simulink model "SnapshotTestBench"  (R2024b)
settings: Solver=VariableStepAuto  StartTime=0.0  StopTime=scenario.StopTime  FixedStep=Ts  RelTol=1e-3
PostLoadFcn:
  | clear all
  | helperSLHighwayLaneChangePlannerSetup
values from neighbouring files (symbols this model uses):
  egoInitialPose = evalin('base','egoInitialPose')    [HelperPlotLCPlannerStatus.m]    (also in HelperPlotLCPlannerStatus_RMC.m; helperSLHighwayLaneChangePlannerSetup.m = struct('ActorID', EgoActor.ActorID,                         )
  mapInfo = struct('NumLanes', numLanes,'LaneWidth', zeros(maxNumLanes,1),                  'LaneCenters', zeros(maxNumLanes,1),'NumGlobalPlanPoints',                  size(globalPlanPoints,1), 'GlobalPlanPoints',                  zeros(maxGlobalPlanPoints,2), 'LaneLateralBoundary', zeros(maxNumLanes, 2))    [helperSLHighwayLaneChangePlannerSetup.m]
  replanRate = 1    [helperSLHighwayLaneChangePlannerSetup.m]
  timeHorizon = 1:3    [helperSLHighwayLaneChangePlannerSetup.m]
  timeResolution = 0.1    [helperSLHighwayLaneChangePlannerSetup.m]
  velocityHorizon = 2    [helperSLHighwayLaneChangePlannerSetup.m]
undefined symbols (not defined in the file or in its folder): ActorID, actorProfiles, AngularVelocity, assessment, egoFrontExt, egoTTC, enableCCBehavior, enableLCBehavior, enableLCFBehavior, frontSafetyGap, latDevCost, maxAccel, maxCurvature, maxPlanningHorizon, maxYawRate, minVelocity, nextTTC, Position, preferredLane, rearSafetyGap, setSpeed, speedCost, targetFrontExt, timeCost, Ts, Velocity, Yaw
libraries: simulink x7, drivingscenarioandsensors x2
CloseFcn:
  | helperSLHighwayLaneChangePlannerCleanUp
settings Model: Creator=The MathWorks, Inc.  LastModifiedBy=grape
settings SolverCC: ZeroCrossAlgorithm=Adaptive  AlgebraicLoopSolver=TrustRegion  MaxZcPerStep=1
settings DataIOCC: SaveOutput=off  ReturnWorkspaceOutputs=off
settings OptimizationCC: ReuseModelBlockBuffer=off  ZeroExternalMemoryAtStartup=off  ZeroInternalMemoryAtStartup=off  OptimizeBlockOrder=speed
settings DebuggingCC: MaskedZcDiagnostic=none  IgnoredZcDiagnostic=none  UnconnectedInputMsg=warning  UnconnectedOutputMsg=warning  UnconnectedLineMsg=warning  SubsystemReferenceDiagnosticForUnitTest=warning
settings ModelReferenceCC: EnableRefExpFcnMdlSchedulingChecks=on
settings RTWCC: Description=Embedded Coder  SystemTargetFile=ert.tlc  TemplateMakefile=ert_default_tmf  PortableWordSizes=on  CodeProfilingSaveOptions=AllData  TargetLang=C++  GPUComputeCapability=3.5  DLArmComputeVersion=19.05
settings CodeAppCC: ForceParamTrailComments=on  IgnoreCustomStorageClasses=off  OperatorAnnotations=on  SimulinkDataObjDesc=on  SFDataObjDesc=on  InsertBlockDesc=on
settings ERTTargetCC: TargetLangStandard=C++03 (ISO)  GenerateSampleERTMain=on  CodeInterfacePackaging=C++ class  InlinedParameterPlacement=Hierarchical  RootIOFormat=Structure reference  ERTCustomFileTemplate=example_file_process.tlc  DynamicArrayContainerType=coder::array
settings ConfigComp: CovScope=ReferencedModels  CovIncludeTopModel=off  CovMetricSettings=dtrzoibwe

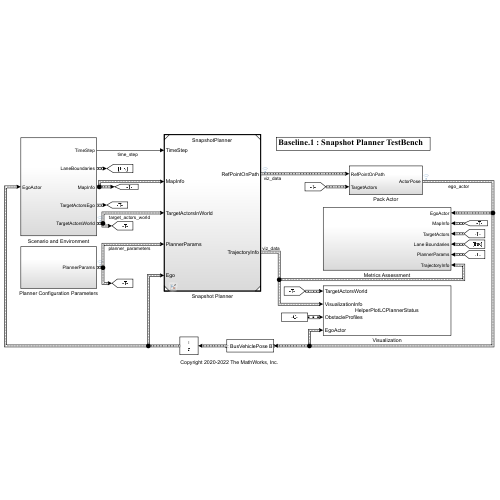
[thumbnail: Simulink's stored preview of the top-level diagram]
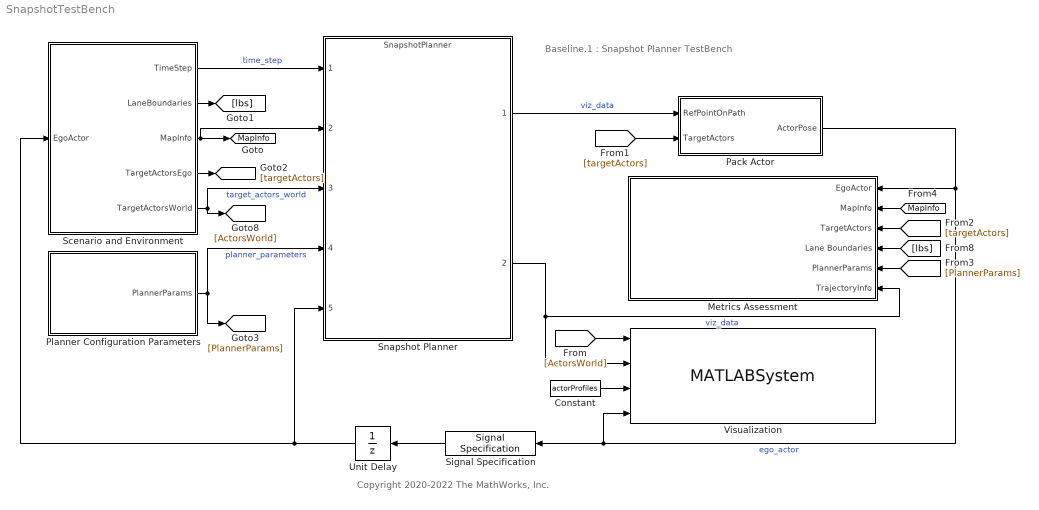
== system SnapshotTestBench ==
  note: Baseline.1 : Snapshot Planner TestBench
  note: Copyright 2020-2022 The MathWorks, Inc.
  Constant : Constant  Value=actorProfiles  OutDataTypeStr=Bus: BusActorProfiles
  Metrics Assessment : Subsystem
  Pack Actor : Subsystem
  Planner Configuration Parameters : Subsystem
  Scenario and Environment : Subsystem
  Signal Specification : SignalSpecification  OutDataTypeStr=Bus: BusVehiclePose  BusOutputAsStruct=on
  Snapshot Planner : ModelReference  ModelNameDialog=SnapshotPlanner.slx  SimulationMode=Normal  ModelReferenceVersion=10.9
  Unit Delay : UnitDelay  InitialCondition=egoInitialPose  SampleTime=-1  HasFrameUpgradeWarning=on
  Visualization : MATLABSystem  System=HelperPlotLCPlannerStatus  EnableTopView=on  EnableTrajTopView=on  EnableChaseView=on  EnableTrajChase=on  EnableCaplistChaseView=on
      mask Type: HelperPlotLCPlannerStatus
      mask Display:
      | disp('HelperPlotLCPlannerStatus');
      | port_label('input',1,'TargetActorsWorld');
      | port_label('input',2,'VisualizationInfo');
      | port_label('input',3,'ObstacleProfiles');
      | port_label('input',4,'EgoActor');
  tag scope: MapInfo=global
  wires:
  Scenario and Environment/4(TargetActorsEgo) -> [targetActors]
  Scenario and Environment/2(LaneBoundaries) -> [lbs]
  Signal Specification/1 -> Unit Delay/1
  [targetActors] -> Pack Actor/2(TargetActors)
  Scenario and Environment/5(TargetActorsWorld) -> Snapshot Planner/3, [ActorsWorld]  "target_actors_world"
  Scenario and Environment/3(MapInfo) -> Snapshot Planner/2, [MapInfo]
  Constant/1 -> Visualization/3
  [ActorsWorld] -> Visualization/1
  Planner Configuration Parameters/1(PlannerParams) -> [PlannerParams], Snapshot Planner/4  "planner_parameters"
  Pack Actor/1(ActorPose) -> Metrics Assessment/1(EgoActor), Visualization/4, Signal Specification/1  "ego_actor"
  Snapshot Planner/2 -> Metrics Assessment/6(TrajectoryInfo), Visualization/2  "viz_data"
  Scenario and Environment/1(TimeStep) -> Snapshot Planner/1  "time_step"
  [targetActors] -> Metrics Assessment/3(TargetActors)
  [lbs] -> Metrics Assessment/4(Lane Boundaries)
  [PlannerParams] -> Metrics Assessment/5(PlannerParams)
  [MapInfo] -> Metrics Assessment/2(MapInfo)
  Snapshot Planner/1 -> Pack Actor/1(RefPointOnPath)  "viz_data"
  Unit Delay/1 -> Scenario and Environment/1(EgoActor), Snapshot Planner/5

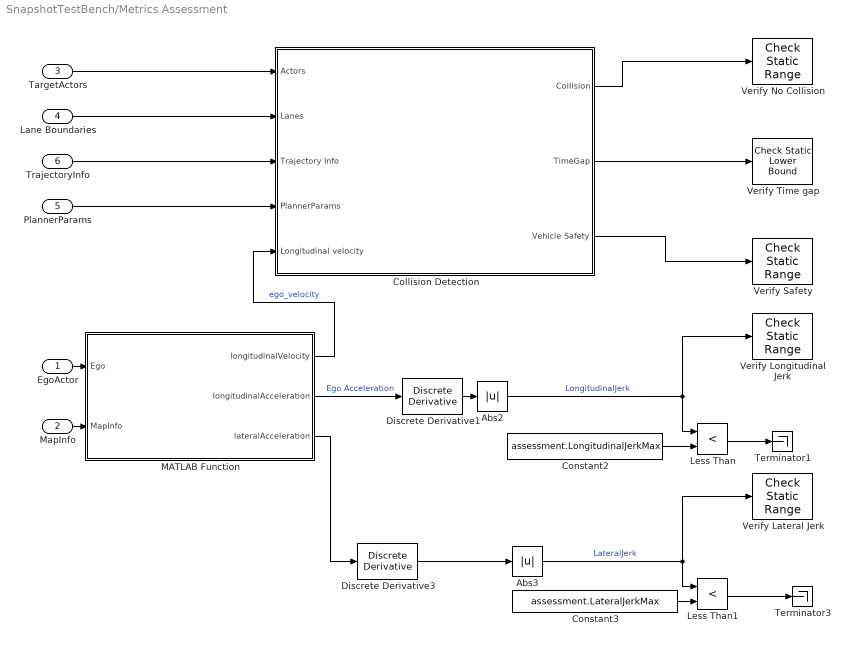
== system SnapshotTestBench/Metrics Assessment ==
  EgoActor : Inport
  MapInfo : Inport  Port=2
  TargetActors : Inport  Port=3
  Lane Boundaries : Inport  Port=4
  PlannerParams : Inport  Port=5
  TrajectoryInfo : Inport  Port=6
  Abs2 : Abs  ZeroCross=off  SaturateOnIntegerOverflow=off
  Abs3 : Abs  ZeroCross=off  SaturateOnIntegerOverflow=off
  Collision Detection : Subsystem
  Constant2 : Constant  Value=assessment.LongitudinalJerkMax
  Constant3 : Constant  Value=assessment.LateralJerkMax
  Discrete Derivative1 : simulink/Discrete/Discrete Derivative  gainval=0.1  ICPrevScaledInput=0.1/Ts  OutMin=[]  OutMax=[]  OutDataType=fixdt(1, 16)  OutScaling=2^-10  DoSatur=off
  Discrete Derivative3 : simulink/Discrete/Discrete Derivative  gainval=0.1  ICPrevScaledInput=0.1/Ts  OutMin=[]  OutMax=[]  OutDataType=fixdt(1, 16)  OutScaling=2^-10  DoSatur=off
  Less Than : RelationalOperator  Operator=<  OutDataTypeStr=boolean  RndMeth=Simplest  InputSameDT=off
  Less Than1 : RelationalOperator  Operator=<  OutDataTypeStr=boolean  RndMeth=Simplest  InputSameDT=off
  MATLAB Function : MATLAB Function  TreatAsAtomicUnit=on
  Terminator1 : Terminator
  Terminator3 : Terminator
  Verify Lateral Jerk : simulink/Model Verification/Check  Static Range  Description=-assessment.LateralJerkMax <= u <= assessment.LateralJerkMax  max=assessment.LateralJerkMax  max_included=on  min=-assessment.LateralJerkMax  min_included=on  enabled=on  stopWhenAssertionFail=off  export=off  icon=graphic
      settings: AttributesFormatString=|
      | ---------------------------------------
      | max = %<max>
      | min = %<min>
  Verify Longitudinal Jerk : simulink/Model Verification/Check  Static Range  Description=-assessment.LongitudinalJerkMax <= u <= assessment.LongitudinalJerkMax  max=assessment.LongitudinalJerkMax  max_included=on  min=-assessment.LongitudinalJerkMax  min_included=on  enabled=on  stopWhenAssertionFail=off  export=off  icon=graphic
      settings: AttributesFormatString=|
      | ---------------------------------------
      | max = %<max>
      | min = %<min>
  Verify No Collision : simulink/Model Verification/Check  Static Range  Description=0 <= u <= 0  max=0  max_included=on  min=0  min_included=on  enabled=on  stopWhenAssertionFail=on  export=off  icon=graphic
  Verify Safety : simulink/Model Verification/Check  Static Range  Description=1 <= u <= 1  max=1  max_included=on  min=1  min_included=on  enabled=on  stopWhenAssertionFail=off  export=off  icon=graphic
  Verify Time gap : simulink/Model Verification/Check Static  Lower Bound  Description=assessment.TimeGap <= u  min=assessment.TimeGap  min_included=on  enabled=on  stopWhenAssertionFail=off  export=off  icon=graphic
      settings: AttributesFormatString=|
      | ---------------------------------------
      | min = %<min>
  wires:
  PlannerParams/1 -> Collision Detection/4(PlannerParams)
  Collision Detection/1(Collision) -> Verify No Collision/1
  Collision Detection/2(TimeGap) -> Verify Time gap/1
  TrajectoryInfo/1 -> Collision Detection/3(Trajectory Info)
  TargetActors/1 -> Collision Detection/1(Actors)
  Collision Detection/3(Vehicle Safety) -> Verify Safety/1
  Lane Boundaries/1 -> Collision Detection/2(Lanes)
  Discrete Derivative1/1 -> Abs2/1
  Discrete Derivative3/1 -> Abs3/1
  Constant3/1 -> Less Than1/2
  Less Than1/1 -> Terminator3/1
  Constant2/1 -> Less Than/2
  Abs2/1 -> Less Than/1, Verify Longitudinal Jerk/1  "LongitudinalJerk"
  Abs3/1 -> Verify Lateral Jerk/1, Less Than1/1  "LateralJerk"
  Less Than/1 -> Terminator1/1
  EgoActor/1 -> MATLAB Function/1(Ego)
  MapInfo/1 -> MATLAB Function/2(MapInfo)
  MATLAB Function/1(longitudinalVelocity) -> Collision Detection/5(Longitudinal velocity)  "ego_velocity"
  MATLAB Function/2(longitudinalAcceleration) -> Discrete Derivative1/1  "Ego Acceleration"
  MATLAB Function/3(lateralAcceleration) -> Discrete Derivative3/1

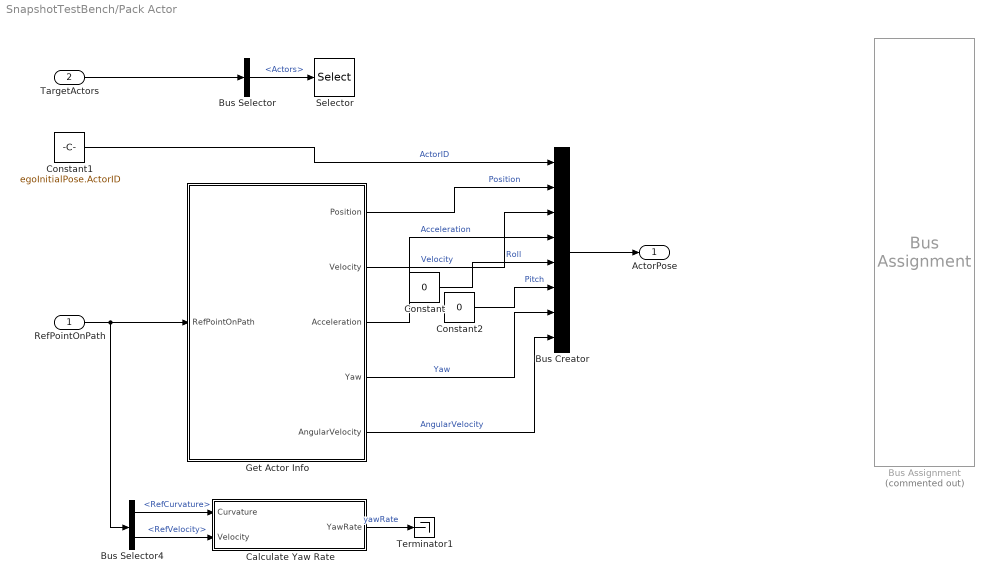
== system SnapshotTestBench/Pack Actor ==
  RefPointOnPath : Inport  SampleTime=Ts
  TargetActors : Inport  Port=2  SampleTime=Ts
  Bus Assignment : BusAssignment  Commented=on  AssignedSignals=ActorID,Position,Velocity,Yaw,AngularVelocity
  Bus Creator : BusCreator  Inputs=8  OutDataTypeStr=Bus: BusVehiclePose  NonVirtualBus=on
  Bus Selector : BusSelector  OutputSignals=Actors
  Bus Selector4 : BusSelector  OutputSignals=RefCurvature,RefVelocity
  Calculate Yaw Rate : MATLAB Function  TreatAsAtomicUnit=on
  Constant : Constant  Value=0
  Constant1 : Constant  Value=egoInitialPose.ActorID
  Constant2 : Constant  Value=0
  Get Actor Info : MATLAB Function  TreatAsAtomicUnit=on
  Selector : Selector  IndexOptions=Index vector (dialog)  Indices=1  OutputSizes=1
  Terminator1 : Terminator
  ActorPose : Outport
  wires:
  RefPointOnPath/1 -> Get Actor Info/1(RefPointOnPath), Bus Selector4/1
  Bus Selector/1 -> Selector/1  "<Actors>"
  TargetActors/1 -> Bus Selector/1
  Bus Selector4/1 -> Calculate Yaw Rate/1(Curvature)  "<RefCurvature>"
  Bus Selector4/2 -> Calculate Yaw Rate/2(Velocity)  "<RefVelocity>"
  Calculate Yaw Rate/1(YawRate) -> Terminator1/1  "yawRate"
  Bus Creator/1 -> ActorPose/1
  Constant1/1 -> Bus Creator/1  "ActorID"
  Get Actor Info/1(Position) -> Bus Creator/2  "Position"
  Get Actor Info/2(Velocity) -> Bus Creator/3  "Velocity"
  Get Actor Info/3(Acceleration) -> Bus Creator/4  "Acceleration"
  Constant/1 -> Bus Creator/5  "Roll"
  Constant2/1 -> Bus Creator/6  "Pitch"
  Get Actor Info/4(Yaw) -> Bus Creator/7  "Yaw"
  Get Actor Info/5(AngularVelocity) -> Bus Creator/8  "AngularVelocity"

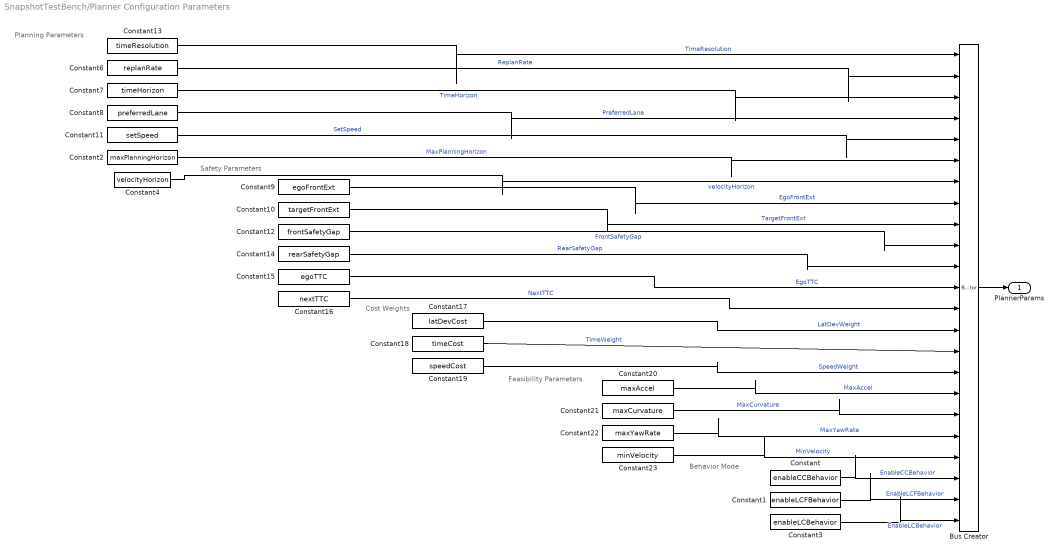
== system SnapshotTestBench/Planner Configuration Parameters ==
  note: Planning Parameters
  note: Safety Parameters
  note: Cost Weights
  note: Feasibility Parameters
  note: Behavior Mode
  Bus Creator : BusCreator  Inputs=23  OutDataTypeStr=Bus: BusPlannerParams  NonVirtualBus=on
  Constant : Constant  Value=enableCCBehavior
  Constant1 : Constant  Value=enableLCFBehavior
  Constant10 : Constant  Value=targetFrontExt
  Constant11 : Constant  Value=setSpeed
  Constant12 : Constant  Value=frontSafetyGap
  Constant13 : Constant  Value=timeResolution
  Constant14 : Constant  Value=rearSafetyGap
  Constant15 : Constant  Value=egoTTC
  Constant16 : Constant  Value=nextTTC
  Constant17 : Constant  Value=latDevCost
  Constant18 : Constant  Value=timeCost
  Constant19 : Constant  Value=speedCost
  Constant2 : Constant  Value=maxPlanningHorizon
  Constant20 : Constant  Value=maxAccel
  Constant21 : Constant  Value=maxCurvature
  Constant22 : Constant  Value=maxYawRate
  Constant23 : Constant  Value=minVelocity
  Constant3 : Constant  Value=enableLCBehavior
  Constant4 : Constant  Value=velocityHorizon
  Constant6 : Constant  Value=replanRate
  Constant7 : Constant  Value=timeHorizon
  Constant8 : Constant  Value=preferredLane
  Constant9 : Constant  Value=egoFrontExt
  PlannerParams : Outport  OutDataTypeStr=Bus: BusPlannerParams
  wires:
  Bus Creator/1 -> PlannerParams/1
  Constant4/1 -> Bus Creator/7  "velocityHorizon"
  Constant3/1 -> Bus Creator/23  "EnableLCBehavior"
  Constant1/1 -> Bus Creator/22  "EnableLCFBehavior"
  Constant/1 -> Bus Creator/21  "EnableCCBehavior"
  Constant23/1 -> Bus Creator/20  "MinVelocity"
  Constant22/1 -> Bus Creator/19  "MaxYawRate"
  Constant21/1 -> Bus Creator/18  "MaxCurvature"
  Constant20/1 -> Bus Creator/17  "MaxAccel"
  Constant19/1 -> Bus Creator/16  "SpeedWeight"
  Constant18/1 -> Bus Creator/15  "TimeWeight"
  Constant17/1 -> Bus Creator/14  "LatDevWeight"
  Constant16/1 -> Bus Creator/13  "NextTTC"
  Constant15/1 -> Bus Creator/12  "EgoTTC"
  Constant14/1 -> Bus Creator/11  "RearSafetyGap"
  Constant12/1 -> Bus Creator/10  "FrontSafetyGap"
  Constant10/1 -> Bus Creator/9  "TargetFrontExt"
  Constant9/1 -> Bus Creator/8  "EgoFrontExt"
  Constant2/1 -> Bus Creator/6  "MaxPlanningHorizon"
  Constant11/1 -> Bus Creator/5  "SetSpeed"
  Constant8/1 -> Bus Creator/4  "PreferredLane"
  Constant7/1 -> Bus Creator/3  "TimeHorizon"
  Constant6/1 -> Bus Creator/2  "ReplanRate"
  Constant13/1 -> Bus Creator/1  "TimeResolution"

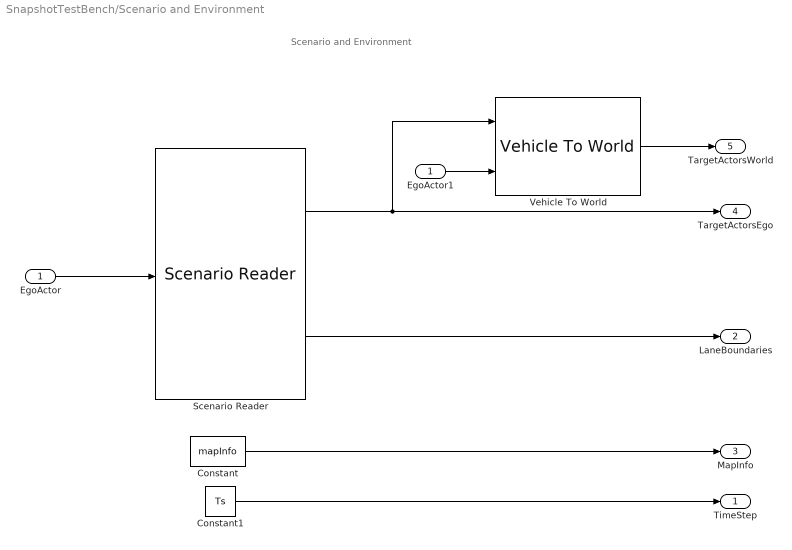
== system SnapshotTestBench/Scenario and Environment ==
  note: Scenario and Environment
  EgoActor : Inport
  Constant : Constant  Value=mapInfo  OutDataTypeStr=Bus: BusMapInfo
  Constant1 : Constant  Value=Ts
  EgoActor1 : InportShadow
  Scenario Reader : drivingscenarioandsensors/Scenario Reader  ScenarioSource=From workspace  ScenarioFileName=CurevedRoadNetwork.mat  ScenarioVariableName=scenario  OutputCoordinateSystem=Vehicle coordinates  EgoVehicleSource=Input port  EgoVehicleActorID=egoInitialPose.ActorID  OrientVehiclesOnRoad=off  OutputEgoVehiclePose=off  OutputEgoVehicleState=off  SampleTime=0.1  LaneBoundaryOutput=Ego vehicle lane boundaries  LaneBoundaryDistance=0:0.5:60  LaneBoundaryLocation=Center of lane markings  BusNameSource=Property  BusName=BusActorsEgo  BusNumActorsSource=Scenario  BusNumActors=100  BusName2Source=Auto  BusName2=BusLaneBoundaries  BusNumLaneBoundariesSource=Scenario  BusNumLaneBoundaries=10  BusName3Source=Auto  BusName3=BusEgoActor  BusName4Source=Auto  BusName4=BusEgoState  ShowCoordinateLabels=on  SimulateUsing=Interpreted execution
  Vehicle To World : drivingscenarioandsensors/Vehicle To World  BusNameSource=Auto  BusName=BusVehicleToWorldActors  SimulateUsing=Interpreted execution
  TimeStep : Outport
  LaneBoundaries : Outport  Port=2
  MapInfo : Outport  Port=3  OutDataTypeStr=Bus: BusMapInfo
  TargetActorsEgo : Outport  Port=4  OutDataTypeStr=Bus: BusActorsEgo  VectorParamsAs1DForOutWhenUnconnected=off
  TargetActorsWorld : Outport  Port=5
  wires:
  EgoActor/1 -> Scenario Reader/1
  Scenario Reader/1 -> Vehicle To World/1, TargetActorsEgo/1
  Scenario Reader/2 -> LaneBoundaries/1
  Constant/1 -> MapInfo/1
  EgoActor1/1 -> Vehicle To World/2
  Vehicle To World/1 -> TargetActorsWorld/1
  Constant1/1 -> TimeStep/1

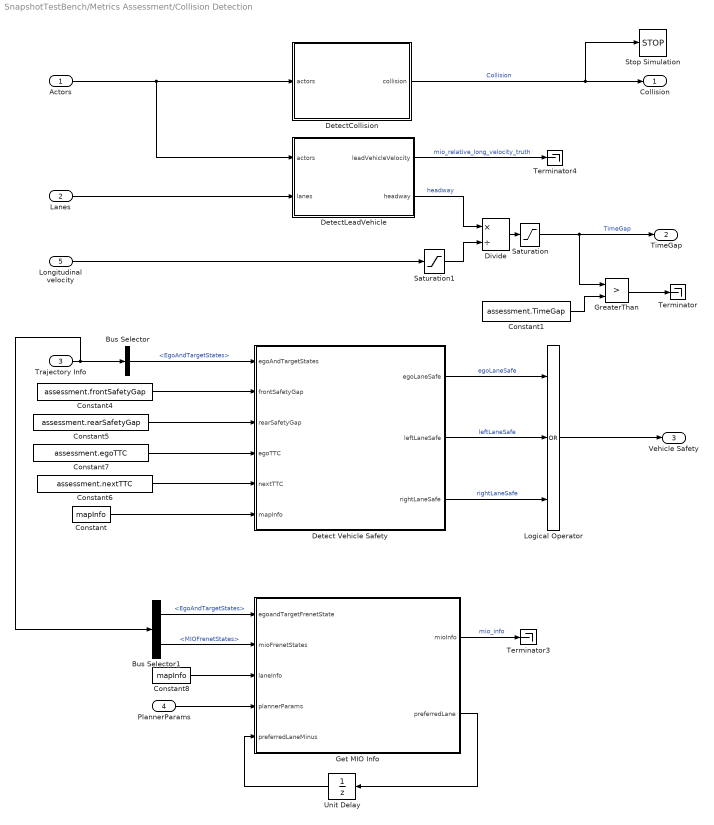
== system SnapshotTestBench/Metrics Assessment/Collision Detection ==
  Actors : Inport
  Lanes : Inport  Port=2
  Trajectory Info : Inport  Port=3
  PlannerParams : Inport  Port=4
  Longitudinal velocity : Inport  Port=5
  Bus Selector : BusSelector  OutputSignals=EgoAndTargetStates
  Bus Selector1 : BusSelector  OutputSignals=EgoAndTargetStates,MIOFrenetStates
  Constant : Constant  Value=mapInfo  OutDataTypeStr=Bus: BusMapInfo
  Constant1 : Constant  Value=assessment.TimeGap
  Constant4 : Constant  Value=assessment.frontSafetyGap
  Constant5 : Constant  Value=assessment.rearSafetyGap
  Constant6 : Constant  Value=assessment.nextTTC
  Constant7 : Constant  Value=assessment.egoTTC
  Constant8 : Constant  Value=mapInfo  OutDataTypeStr=Bus: BusMapInfo
  Detect Vehicle Safety : MATLAB Function  TreatAsAtomicUnit=on
  DetectCollision : MATLAB Function  TreatAsAtomicUnit=on  mask{actorProfile=actorProfiles, egoActorID=egoInitialPose.ActorID}
      mask prompts: actorProfile "ActorProfiles"
  DetectLeadVehicle : MATLAB Function  TreatAsAtomicUnit=on  mask{vehicleProfiles=actorProfiles}
      mask prompts: vehicleProfiles "Vehicle profiles"
  Divide : Product  Inputs=*/
  Get MIO Info : MATLAB Function  TreatAsAtomicUnit=on  mask{outputStructObj=Simulink.Bus.createMATLABStruct('BusMIOInfo')}
      mask prompts: outputStructObj "Output Structure"
  GreaterThan : RelationalOperator  Operator=>  OutDataTypeStr=boolean  RndMeth=Simplest  InputSameDT=off
  Logical Operator : Logic  Operator=OR  Inputs=3  AllPortsSameDT=off  OutDataTypeStr=boolean
  Saturation : Saturate  UpperLimit=4  LowerLimit=0
  Saturation1 : Saturate  UpperLimit=100  LowerLimit=0.01
  Stop Simulation : Stop
  Terminator : Terminator
  Terminator3 : Terminator
  Terminator4 : Terminator
  Unit Delay : UnitDelay  SampleTime=-1  HasFrameUpgradeWarning=on
  Collision : Outport
  TimeGap : Outport  Port=2
  Vehicle Safety : Outport  Port=3
  wires:
  Divide/1 -> Saturation/1
  Actors/1 -> DetectCollision/1(actors), DetectLeadVehicle/1(actors)
  DetectCollision/1(collision) -> Stop Simulation/1, Collision/1  "Collision"
  Saturation1/1 -> Divide/2
  DetectLeadVehicle/2(headway) -> Divide/1  "headway"
  DetectLeadVehicle/1(leadVehicleVelocity) -> Terminator4/1  "mio_relative_long_velocity_truth"
  Saturation/1 -> GreaterThan/1, TimeGap/1  "TimeGap"
  Constant1/1 -> GreaterThan/2
  Lanes/1 -> DetectLeadVehicle/2(lanes)
  GreaterThan/1 -> Terminator/1
  Longitudinal velocity/1 -> Saturation1/1
  Constant6/1 -> Detect Vehicle Safety/5(nextTTC)
  Bus Selector/1 -> Detect Vehicle Safety/1(egoAndTargetStates)  "<EgoAndTargetStates>"
  Constant5/1 -> Detect Vehicle Safety/3(rearSafetyGap)
  Logical Operator/1 -> Vehicle Safety/1
  Constant/1 -> Detect Vehicle Safety/6(mapInfo)
  Constant7/1 -> Detect Vehicle Safety/4(egoTTC)
  Detect Vehicle Safety/3(rightLaneSafe) -> Logical Operator/3  "rightLaneSafe"
  Constant4/1 -> Detect Vehicle Safety/2(frontSafetyGap)
  Detect Vehicle Safety/1(egoLaneSafe) -> Logical Operator/1  "egoLaneSafe"
  Detect Vehicle Safety/2(leftLaneSafe) -> Logical Operator/2  "leftLaneSafe"
  Get MIO Info/2(preferredLane) -> Unit Delay/1
  PlannerParams/1 -> Get MIO Info/4(plannerParams)
  Get MIO Info/1(mioInfo) -> Terminator3/1  "mio_info"
  Unit Delay/1 -> Get MIO Info/5(preferredLaneMinus)
  Bus Selector1/1 -> Get MIO Info/1(egoandTargetFrenetState)  "<EgoAndTargetStates>"
  Trajectory Info/1 -> Bus Selector1/1, Bus Selector/1
  Bus Selector1/2 -> Get MIO Info/2(mioFrenetStates)  "<MIOFrenetStates>"
  Constant8/1 -> Get MIO Info/3(laneInfo)

== matlab function SnapshotTestBench/Pack Actor/Calculate Yaw Rate ==
  data: Curvature input; YawRate output; Velocity input
function YawRate = calculateYawRate(Curvature, Velocity)
    YawRate = Curvature.*Velocity;
end

== matlab function SnapshotTestBench/Metrics Assessment/MATLAB Function ==
  data: Ego input; longitudinalVelocity output; MapInfo input; longitudinalAcceleration output; lateralAcceleration output
function [longitudinalVelocity, longitudinalAcceleration, lateralAcceleration] = egoFrenetStateConverter(Ego, MapInfo)

persistent RefPathFrenet 
refPath = MapInfo.GlobalPlanPoints(1:MapInfo.NumGlobalPlanPoints,:);
if isempty(RefPathFrenet)    
    RefPathFrenet = referencePathFrenet(refPath);   
else
    %Check for a change in the reference path
    if ~isequal(RefPathFrenet.Waypoints, refPath) 
        refPathNew = referencePathFrenet(refPath);
        RefPathFrenet.Waypoints = refPathNew.Waypoints;
    end
end

kappa = deg2rad(Ego.AngularVelocity(3))/norm(Ego.Velocity);
if (isnan(kappa) || isinf(kappa))
    kappa = 0;
end
egoState = [Ego.Position(1:2), deg2rad(Ego.Yaw), kappa, norm(Ego.Velocity(1:2),2), 0]; 

egoFrenetState = global2frenet(RefPathFrenet, egoState); % [S dS ddS L dL ddL]

longitudinalVelocity = egoFrenetState(2);
longitudinalAcceleration = egoFrenetState(3); % ddS/ddt
lateralAcceleration = egoFrenetState(6) * longitudinalAcceleration; % ddL/ddS * ddS/ddt = ddL/ddt
% [S dS ddS L dL ddL], where S is the arc length and L is the perpendicular
% deviation from the direction of the reference path. Derivatives of S are
% relative to time. Derivatives of L are relative to the arc length, S.

== matlab function SnapshotTestBench/Pack Actor/Get Actor Info ==
  data: RefPointOnPath input; Position output; Velocity output; Acceleration output; Yaw output; AngularVelocity output
function [Position, Velocity, Acceleration, Yaw, AngularVelocity] = GetActorInfo(RefPointOnPath)
%GetActorInfo function extracts the information required for actor bus
%information.
%
% This function outputs position, velocity, Yaw angle and angular velocity
% of the ego vehicle. This information is used to update the actor bus.

% Get Position vector
Position = [RefPointOnPath.RefPoseRr(1:2) 0];

% Get orientation of the actor
Yaw = RefPointOnPath.RefPoseRr(3);

% Get Velocity vector
velocity = RefPointOnPath.RefVelocity;
Velocity = [velocity*cosd(Yaw) velocity*sind(Yaw) 0];

accel = RefPointOnPath.RefAccel;
Acceleration = [accel*cosd(Yaw), accel*sind(Yaw), 0];

% Get Angular velocity
AngularVelocity = [0 0 RefPointOnPath.RefAngVel];

end

== matlab function SnapshotTestBench/Metrics Assessment/Collision Detection/Detect Vehicle Safety ==
  data: egoAndTargetStates input; egoLaneSafe output; frontSafetyGap input; rearSafetyGap input; egoTTC input; nextTTC input; mapInfo input; leftLaneSafe output; rightLaneSafe output
function [egoLaneSafe, leftLaneSafe, rightLaneSafe]  = vehicleSafetyDetection(egoAndTargetStates, frontSafetyGap, rearSafetyGap, egoTTC, nextTTC, mapInfo)

egoFrenetState = egoAndTargetStates.EgoFrenetState;

numTargets = egoAndTargetStates.NumTargetActors;
targetFrenetStates = egoAndTargetStates.TargetFrenetStates(1:numTargets, :);

curEgoLane = helperDetectLaneNumber(mapInfo,egoFrenetState(4));

targetLanes = zeros(numTargets,1);
targetTTCs = zeros(numTargets,1);
targetRanges = zeros(numTargets,1);
targetVels = zeros(numTargets,1);
targetFront = zeros(numTargets,1);
mioSafe = zeros(numTargets,1);
% egoLaneSafe = 0;
leftLaneSafe = false;
rightLaneSafe = false;
for i = 1:numTargets
        % Get MIO lane
        targetLanes(i) = helperDetectLaneNumber(mapInfo, targetFrenetStates(i,4));        
        
        % Calculate TTC and other attributes of MIOs with ego vehicle
        [targetRanges(i),~,targetVels(i),targetTTCs(i),targetFront(i)] = helperCalculateTTC(egoFrenetState,targetFrenetStates(i,:));
        mioSafe(i) = checkSafety(targetLanes(i),targetRanges(i),targetTTCs(i),targetFront(i),curEgoLane,frontSafetyGap, rearSafetyGap, egoTTC,nextTTC);        
end

% check ego lane
egoLane = targetLanes==curEgoLane;
% disp(mioSafe(egoLane));
egoLaneSafe = isempty(mioSafe(egoLane)) || all(mioSafe(egoLane));

% check left lane
leftLane = targetLanes==(curEgoLane-1);
if curEgoLane>1
    leftLaneSafe = (isempty(mioSafe(leftLane)) || all(mioSafe(leftLane))); 
end

% check right lane
rightLane = targetLanes==(curEgoLane+1);
if curEgoLane<mapInfo.NumLanes 
    rightLaneSafe = (isempty(mioSafe(rightLane)) || all(mioSafe(rightLane)));
end
end
function isSafe = checkSafety(Lane,Range,TTC,Front,EgoLane,frontSafetyGap,rearSafetyGap,egoTTC,nextTTC)
%checkSafety function checks for safety of current ego lane, and it's
%adjacent lanes.

% default: current lane is unsafe
isSafe = true;

if Front
    SafetyGap = frontSafetyGap;
else
    SafetyGap = rearSafetyGap;
end

if Lane==EgoLane % ego lane
    if Range < SafetyGap || ... % mio is too close?
            (TTC < 0 && ... % mio is approaching
            abs(TTC) < egoTTC) % TTC is too small?
        isSafe = false; % current lane is unsafe
    end
else % left or right lane
    if Range < SafetyGap || ... % mio is too close?
            (TTC < 0 && ... % mio is approaching
            abs(TTC) < nextTTC) % TTC is too small?
        isSafe = false; % current lane is unsafe
    end   
end

end

== matlab function SnapshotTestBench/Metrics Assessment/Collision Detection/DetectCollision ==
  data: actors input; collision output; actorProfile parameter; egoActorID parameter
%% collisionDetect
% Detects if there is any collision while running the model.
function collision  = collisionDetect(actors, actorProfile, egoActorID)
coder.extrinsic('area');
coder.extrinsic('intersect');
coder.extrinsic('union');

egoActor.Position = [0 0];
egoActor.Yaw = 0;
p1 = vehicle2polyshape(egoActor,1.8,4.7,1,[1 0.1]);

collision = false;

overlapRatio = double(0);
actorIdx = 1;
for i = 1:numel(actorProfile)
    if actorProfile(i).ActorID ~= egoActorID
        w = actorProfile(i).Width;
        h = actorProfile(i).Length;
        RO = actorProfile(i).Length * 0.5 + actorProfile(i).OriginOffset(1);
        p2 = vehicle2polyshape(actors.Actors(actorIdx),w,h,RO,[0 0]);
        
        overlapRatio = area(intersect(p1,p2))/area(union(p1,p2));
        
        if overlapRatio > 0.01
            collision = true; % collision detected
            return;
        end
        actorIdx = actorIdx + 1;
    end
end

end

function pshape = vehicle2polyshape(vehicle,w,h,RO,margin)
% vehicle.Position : position (x,y) of vehicle
% vehicle.Yaw : orientation of vehicle
% w: width
% h: height
% RO: read overhang

coder.extrinsic('polyshape');
coder.extrinsic('rotate');

x = vehicle.Position(1);
y = vehicle.Position(2);
theta = vehicle.Yaw - 90;

xcoord = [x-w/2-margin(2), x+w/2+margin(2), x+w/2+margin(2), x-w/2-margin(2)];
ycoord = [y-RO-margin(1), y-RO-margin(1), y+h-RO+margin(1), y+h-RO+margin(1)];
pshape = rotate(polyshape(xcoord, ycoord), theta, [x, y]);
end

== matlab function SnapshotTestBench/Metrics Assessment/Collision Detection/DetectLeadVehicle ==
  data: leadVehicleVelocity output; actors input; headway output; lanes input; vehicleProfiles parameter
function [leadVehicleVelocity, headway]  = detectLeadVehicle(actors, lanes,vehicleProfiles)

% Find the closest vehicle in ego lane
longDist = zeros(1,actors.NumActors);


for i = 1:actors.NumActors
    
    % Positions of the actor with respect to ego in X-direction
    x = actors.Actors(i).Position(1);
    y = actors.Actors(i).Position(2);
    
    % Default longitudinal distance from vehicle
    longDist(i) = inf;
    
    % Check if vehicle is ahead of ego
    if x >= 0
        % Find left lane coordinates closest to vehicle position x
        [~,n] = min(abs(lanes.LaneBoundaries(1).Coordinates(:,1)-x));
        yleftLane = lanes.LaneBoundaries(1).Coordinates(n,2);

        % Find right lane coordinates closest to vehicle position x
        [~,n] = min(abs(lanes.LaneBoundaries(2).Coordinates(:,1)-x));
        yrightLane = lanes.LaneBoundaries(2).Coordinates(n,2);

        % Check if vehicle is in same lane as ego
        if (yrightLane <= y) && (y <= yleftLane)
            longDist(i) = x;
        end       
    end
end
% Minimum distance between vehicle rear axles
[minLongDist,mioIndex] = min(longDist);

% Get lead vehicle information
if isempty(minLongDist) || isinf(minLongDist)
    headway = inf;
    leadVehicleVelocity = inf;
else
    headway = headwayLongDist(minLongDist,mioIndex,vehicleProfiles);
    leadVehicleVelocity = norm(actors.Actors(mioIndex).Velocity);
end

end

function headway = headwayLongDist(dist,mioIndex,vehicleProfiles)
% Longitudinal headway is distance between vehicle rear axles
% reduced by distance of ego rear axle to front and 
% reduced by distance of MIO rear axle to rear

% Notes on origin offset
% - Origin offset is the relative position [x,yz] of vehicle center with 
%   respect to the rear axle
% - Distance rear axle center to vehicle center = negative of origin offset(1)

% Ego distance from rear axle to front
egoProfile = vehicleProfiles(1);
egoDistRearAxleToVehCenter = - egoProfile.OriginOffset(1);
egoDistRearAxleToFront = egoProfile.Length/2 + egoDistRearAxleToVehCenter;

% MIO distance from rear axle to rear
mioProfile = vehicleProfiles(mioIndex);
mioDistRearAxleToVehCenter = - mioProfile.OriginOffset(1);
mioDistRearAxleToRear = mioProfile.Length/2 - mioDistRearAxleToVehCenter;

% Longitudinal headway is distance from front of ego to rear of MIO
headway = dist - egoDistRearAxleToFront - mioDistRearAxleToRear;

end

== matlab function SnapshotTestBench/Metrics Assessment/Collision Detection/Get MIO Info ==
  data: mioInfo output Bus: BusMIOInfo; egoandTargetFrenetState input; preferredLane output; mioFrenetStates input; laneInfo input; plannerParams input; preferredLaneMinus input; outputStructObj parameter
function [mioInfo, preferredLane] = getMIOInfo(egoandTargetFrenetState,...
                                               mioFrenetStates, laneInfo,...
                                               plannerParams,...
                                               preferredLaneMinus,...
                                               outputStructObj)


% Get ego actor frenet states from EgoAndTargetStates bus structure
egoFrenetState = egoandTargetFrenetState.EgoFrenetState;

[preferredLane, mioInfo]= helperFindPreferredLane(egoFrenetState,...
                                                  mioFrenetStates,...
                                                  laneInfo,plannerParams,...
                                                  preferredLaneMinus,...
                                                  outputStructObj);

end
